simulink model "VD_L_filter"  (R2018b)
settings: Solver=ode8  StartTime=0.0  StopTime=1  RelTol=1e-3
undefined symbols (not defined in the file): C, L, Rn
libraries: powerlib x16, powerlib_meascontrol x8, peRmsMeasurement x4
settings Model: Creator=Anton  LastModifiedBy=VID Company
settings SFSimCC: SimUseLocalCustomCode=off
settings RTWCC: RTWUseLocalCustomCode=off
settings CodeAppCC: StateflowObjectComments=on
settings SimscapeCC: SimscapeNormalizeSystem=off

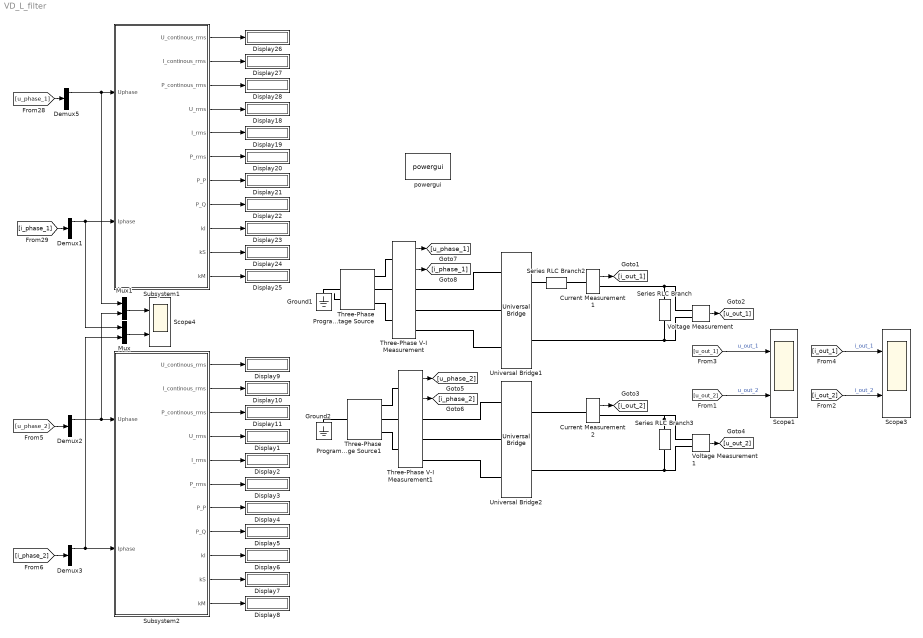
== system VD_L_filter ==
  Current Measurement1 : powerlib/Measurements/Current Measurement  PhasorSimulation=off  OutputType=Complex  PSBequivalent=0
  Current Measurement2 : powerlib/Measurements/Current Measurement  PhasorSimulation=off  OutputType=Complex  PSBequivalent=0
  Demux{1..3,5} (4 alike) : Demux  Outputs=3
  Display{1..11,18..28} (22 alike) : Display
  Ground1 : powerlib/Elements/Ground  LConnTagsString=a
  Ground2 : powerlib/Elements/Ground  LConnTagsString=a
  Mux : Mux  Inputs=2
  Mux1 : Mux  Inputs=2
  Scope1 : Scope  NumInputPorts=2
  Scope3 : Scope  NumInputPorts=2
  Scope4 : Scope  NumInputPorts=2
  Series RLC Branch : powerlib/Elements/Series RLC Branch  LConnTagsString=__new0  RConnTagsString=__new0  BranchType=R  Resistance=Rn  Inductance=250e-6  SetiL0=off  InitialCurrent=0  Capacitance=1e-6  Setx0=off  InitialVoltage=0  Measurements=None
  Series RLC Branch2 : powerlib/Elements/Series RLC Branch  LConnTagsString=__new0  RConnTagsString=__new0  BranchType=L  Resistance=1e-3  Inductance=L  SetiL0=off  InitialCurrent=0  Capacitance=C  Setx0=on  InitialVoltage=Un  Measurements=None
  Series RLC Branch3 : powerlib/Elements/Series RLC Branch  LConnTagsString=__new0  RConnTagsString=__new0  BranchType=R  Resistance=Rn  Inductance=250e-6  SetiL0=off  InitialCurrent=0  Capacitance=1e-6  Setx0=off  InitialVoltage=0  Measurements=None
  Subsystem1 : Subsystem
  Subsystem2 : Subsystem
  Three-Phase Programmable Voltage Source : powerlib/Electrical Sources/Three-Phase Programmable Voltage Source  PositiveSequence=[390 0 50]  VariationEntity=None  VariationType=Table of time-amplitude pairs  VariationTypeAlt=Step  VariationStep=0.5  VariationRate=10  VariationMagnitude=0.3  VariationFrequency=2  VariationTiming=[1 2]  VariationPhaseA=off  Amplitudes=[1 0.8 1.2 1.0]  TimeValues=[0 0.1 0.15 0.2]  HarmonicGeneration=off  HarmonicA=[3 0.2 -25 0]  HarmonicB=[2 0.15 35 2]  Timing="[0.05  3]"  BusType=swing  Pref=0  Qref=0  Qmin=-inf  Qmax=inf
  Three-Phase Programmable Voltage Source1 : powerlib/Electrical Sources/Three-Phase Programmable Voltage Source  PositiveSequence=[390 0 50]  VariationEntity=None  VariationType=Table of time-amplitude pairs  VariationTypeAlt=Step  VariationStep=0.5  VariationRate=10  VariationMagnitude=0.3  VariationFrequency=2  VariationTiming=[1 2]  VariationPhaseA=off  Amplitudes=[1 0.8 1.2 1.0]  TimeValues=[0 0.1 0.15 0.2]  HarmonicGeneration=off  HarmonicA=[3 0.2 -25 0]  HarmonicB=[2 0.15 35 2]  Timing="[0.05  3]"  BusType=swing  Pref=0  Qref=0  Qmin=-inf  Qmax=inf
  Three-Phase V-I Measurement : powerlib/Measurements/Three-Phase V-I Measurement  VoltageMeasurement=phase-to-ground  SetLabelV=off  LabelV=Vabc  Vpu=off  VpuLL=off  CurrentMeasurement=yes  SetLabelI=off  LabelI=Iabc  Ipu=off  Pbase=100e6  Vbase=500e3  OutputType=Complex  PhasorSimulation=off  PSBequivalent=0
  Three-Phase V-I Measurement1 : powerlib/Measurements/Three-Phase V-I Measurement  VoltageMeasurement=phase-to-ground  SetLabelV=off  LabelV=Vabc  Vpu=off  VpuLL=off  CurrentMeasurement=yes  SetLabelI=off  LabelI=Iabc  Ipu=off  Pbase=100e6  Vbase=500e3  OutputType=Complex  PhasorSimulation=off  PSBequivalent=0
  Universal Bridge1 : powerlib/Power Electronics/Universal Bridge  Arms=3  SnubberResistance=1e5  SnubberCapacitance=inf  Device=Diodes  Ron=1e-3  Lon=0  ForwardVoltages="[  0  0  ]"  ForwardVoltage=1  GTOparameters=[ 10e-6 , 20e-6 ]  IGBTparameters=[ 1e-6 , 2e-6 ]  Measurements=None  Measurements_2=None  converterType=Rectifier
  Universal Bridge2 : powerlib/Power Electronics/Universal Bridge  Arms=3  SnubberResistance=1e5  SnubberCapacitance=inf  Device=Diodes  Ron=1e-9  Lon=0  ForwardVoltages="[  0  0  ]"  ForwardVoltage=1  GTOparameters=[ 10e-6 , 20e-6 ]  IGBTparameters=[ 1e-6 , 2e-6 ]  Measurements=None  Measurements_2=None  converterType=Rectifier
  Voltage Measurement : powerlib/Measurements/Voltage Measurement  PhasorSimulation=off  OutputType=Complex  PSBequivalent=0
  Voltage Measurement1 : powerlib/Measurements/Voltage Measurement  PhasorSimulation=off  OutputType=Complex  PSBequivalent=0
  powergui : powerlib/powergui  Priority=1  SimulationMode=Discrete  SampleTime=1e-6  frequency=60  Iterations=50  frequencyindice=0  Pbase=100e6  ErrMax=1e-4  UnitsV=kV  UnitsW=MW  buscounter=0  FunctionMessages=off  echomessages=off  EnableUseOfTLC=off  CurrentSourceSwitches=off  DisableSnubberDevices=off  DisableRonSwitches=off  DisableVfSwitches=off  DisplayEquations=off  SolverType=Tustin/Backward Euler (TBE)  Interpol=off  ExternalGateDelay=off  methode=off  Ts=100  x0status=blocks  SPID=off  SwTol=0  HookPort=off  RestoreLinks=warning  ResistiveCurrentMeasurement=off  Frange=[0:2:500]  Ylog=off  Xlog=on  ShowGrid=off  save=off  variable=ZData  structure=0  ZoomFFT=off  StartTime=0.0  cycles=1  DisplayStyle=1  fundamental=60  FreqAxis=off  MaxFrequency=1000  frequencyindicesteady=1  RmsSteady=1  display=off
  wires:
  Three-Phase V-I Measurement/2 -> [i_phase_1]
  Three-Phase V-I Measurement/1 -> [u_phase_1]
  Voltage Measurement/1 -> [u_out_1]
  Current Measurement1/1 -> [i_out_1]
  Current Measurement2/1 -> [i_out_2]
  Voltage Measurement1/1 -> [u_out_2]
  [u_out_1] -> Scope1/1  "u_out_1"
  [u_out_2] -> Scope1/2  "u_out_2"
  [i_out_1] -> Scope3/1  "i_out_1"
  [i_out_2] -> Scope3/2  "i_out_2"
  Subsystem1/8(P_Q) -> Display22/1
  Subsystem1/2(I_continous_rms) -> Display27/1
  Subsystem1/7(P_P) -> Display21/1
  Subsystem1/4(U_rms) -> Display18/1
  Subsystem1/3(P_continous_rms) -> Display28/1
  Subsystem1/9(kI) -> Display23/1
  Subsystem1/11(kM) -> Display25/1
  Subsystem1/6(P_rms) -> Display20/1
  Subsystem1/10(kS) -> Display24/1
  Subsystem1/5(I_rms) -> Display19/1
  Subsystem1/1(U_continous_rms) -> Display26/1
  Three-Phase V-I Measurement1/1 -> [u_phase_2]
  Three-Phase V-I Measurement1/2 -> [i_phase_2]
  Mux/1 -> Scope4/2
  Mux1/1 -> Scope4/1
  [u_phase_1] -> Demux5/1
  Demux5/1 -> Mux1/1, Subsystem1/1(Uphase)
  [i_phase_1] -> Demux1/1
  Demux1/1 -> Mux/1, Subsystem1/2(Iphase)
  Subsystem2/10(kS) -> Display7/1
  Subsystem2/6(P_rms) -> Display3/1
  Subsystem2/1(U_continous_rms) -> Display9/1
  Subsystem2/5(I_rms) -> Display2/1
  Subsystem2/9(kI) -> Display6/1
  Subsystem2/4(U_rms) -> Display1/1
  Subsystem2/3(P_continous_rms) -> Display11/1
  Subsystem2/7(P_P) -> Display4/1
  Subsystem2/11(kM) -> Display8/1
  Subsystem2/2(I_continous_rms) -> Display10/1
  Subsystem2/8(P_Q) -> Display5/1
  Demux2/1 -> Mux1/2, Subsystem2/1(Uphase)
  [u_phase_2] -> Demux2/1
  Demux3/1 -> Mux/2, Subsystem2/2(Iphase)
  [i_phase_2] -> Demux3/1
  connections:
  Universal Bridge1/LConn1 -- Three-Phase V-I Measurement/RConn1
  Universal Bridge1/LConn3 -- Three-Phase V-I Measurement/RConn3
  Universal Bridge1/LConn2 -- Three-Phase V-I Measurement/RConn2
  Three-Phase Programmable Voltage Source/RConn1 -- Three-Phase V-I Measurement/LConn1
  Three-Phase Programmable Voltage Source/LConn1 -- Ground1/LConn1
  Three-Phase Programmable Voltage Source/RConn3 -- Three-Phase V-I Measurement/LConn3
  Three-Phase Programmable Voltage Source/RConn2 -- Three-Phase V-I Measurement/LConn2
  Series RLC Branch/RConn1 -- Universal Bridge1/RConn2 -- Voltage Measurement/LConn2
  Voltage Measurement/LConn1 -- Current Measurement1/RConn1 -- Series RLC Branch/LConn1
  Current Measurement1/LConn1 -- Series RLC Branch2/RConn1
  Voltage Measurement1/LConn2 -- Series RLC Branch3/RConn1 -- Universal Bridge2/RConn2
  Series RLC Branch3/LConn1 -- Voltage Measurement1/LConn1 -- Current Measurement2/RConn1
  Current Measurement2/LConn1 -- Universal Bridge2/RConn1
  Universal Bridge2/LConn2 -- Three-Phase V-I Measurement1/RConn2
  Three-Phase Programmable Voltage Source1/RConn3 -- Three-Phase V-I Measurement1/LConn3
  Three-Phase Programmable Voltage Source1/RConn1 -- Three-Phase V-I Measurement1/LConn1
  Three-Phase Programmable Voltage Source1/LConn1 -- Ground2/LConn1
  Three-Phase Programmable Voltage Source1/RConn2 -- Three-Phase V-I Measurement1/LConn2
  Universal Bridge2/LConn1 -- Three-Phase V-I Measurement1/RConn1
  Universal Bridge2/LConn3 -- Three-Phase V-I Measurement1/RConn3
  Series RLC Branch2/LConn1 -- Universal Bridge1/RConn1
  ?

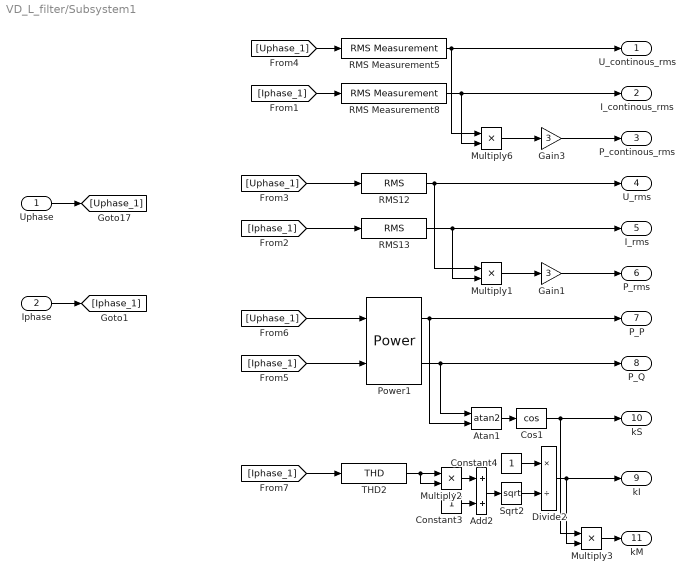
== system VD_L_filter/Subsystem1 ==
  Uphase : Inport
  Iphase : Inport  Port=2
  Add2 : Sum
  Atan1 : Trigonometry  Operator=atan2
  Constant3 : Constant
  Constant4 : Constant
  Cos1 : Trigonometry  Operator=cos
  Divide2 : Product  Inputs=*/
  Gain1 : Gain  Gain=3
  Gain3 : Gain  Gain=3
  Multiply{1..3,6} (4 alike) : Product
  Power1 : powerlib_meascontrol/Measurements/Power  Freq=50  Vinit=[1, 0]  Iinit=[1, 0]  Ts=0
      settings: SourceProductName=Simscape Power Systems
  RMS Measurement5 : peRmsMeasurement/RMS Measurement  LabelModeActiveChoice=Harmonic  F=50  SpecifyHarmonics=on  K=[1]  Ts=0
  RMS Measurement8 : peRmsMeasurement/RMS Measurement  LabelModeActiveChoice=Harmonic  F=50  SpecifyHarmonics=on  K=[1]  Ts=0
  RMS12 : powerlib_meascontrol/Measurements/RMS  TrueRMS=on  Freq=50  RMSInit=0  Ts=0
  RMS13 : powerlib_meascontrol/Measurements/RMS  TrueRMS=on  Freq=50  RMSInit=0  Ts=0
  Sqrt2 : Sqrt  SaturateOnIntegerOverflow=on
  THD2 : powerlib_meascontrol/Measurements/THD  Freq=50  Ts=0
  U_continous_rms : Outport
  I_continous_rms : Outport  Port=2
  P_continous_rms : Outport  Port=3
  U_rms : Outport  Port=4
  I_rms : Outport  Port=5
  P_rms : Outport  Port=6
  P_P : Outport  Port=7
  P_Q : Outport  Port=8
  kI : Outport  Port=9
  kS : Outport  Port=10
  kM : Outport  Port=11
  wires:
  RMS Measurement5/1 -> Multiply6/1, U_continous_rms/1
  RMS Measurement8/1 -> Multiply6/2, I_continous_rms/1
  [Uphase_1] -> RMS Measurement5/1
  [Iphase_1] -> RMS Measurement8/1
  Multiply6/1 -> Gain3/1
  RMS12/1 -> Multiply1/1, U_rms/1
  [Uphase_1] -> RMS12/1
  [Iphase_1] -> RMS13/1
  RMS13/1 -> Multiply1/2, I_rms/1
  Multiply1/1 -> Gain1/1
  Atan1/1 -> Cos1/1
  Power1/1 -> Atan1/2, P_P/1
  Power1/2 -> Atan1/1, P_Q/1
  [Uphase_1] -> Power1/1
  [Iphase_1] -> Power1/2
  Cos1/1 -> Multiply3/1, kS/1
  Sqrt2/1 -> Divide2/2
  THD2/1 -> Multiply2/1, Multiply2/2
  Constant3/1 -> Add2/2
  Multiply2/1 -> Add2/1
  Constant4/1 -> Divide2/1
  Divide2/1 -> Multiply3/2, kI/1
  Add2/1 -> Sqrt2/1
  [Iphase_1] -> THD2/1
  Multiply3/1 -> kM/1
  Gain3/1 -> P_continous_rms/1
  Gain1/1 -> P_rms/1
  Uphase/1 -> [Uphase_1]
  Iphase/1 -> [Iphase_1]

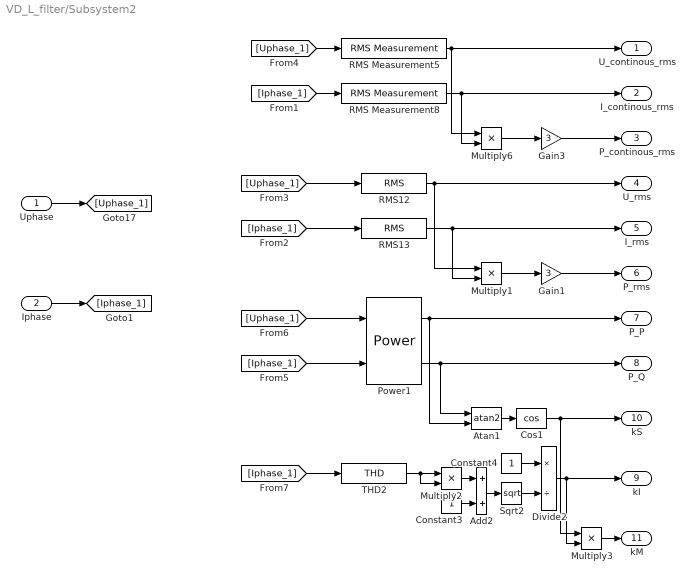
== system VD_L_filter/Subsystem2 ==
  Uphase : Inport
  Iphase : Inport  Port=2
  Add2 : Sum
  Atan1 : Trigonometry  Operator=atan2
  Constant3 : Constant
  Constant4 : Constant
  Cos1 : Trigonometry  Operator=cos
  Divide2 : Product  Inputs=*/
  Gain1 : Gain  Gain=3
  Gain3 : Gain  Gain=3
  Multiply{1..3,6} (4 alike) : Product
  Power1 : powerlib_meascontrol/Measurements/Power  Freq=50  Vinit=[1, 0]  Iinit=[1, 0]  Ts=0
      settings: SourceProductName=Simscape Power Systems
  RMS Measurement5 : peRmsMeasurement/RMS Measurement  LabelModeActiveChoice=Harmonic  F=50  SpecifyHarmonics=on  K=[1]  Ts=0
  RMS Measurement8 : peRmsMeasurement/RMS Measurement  LabelModeActiveChoice=Harmonic  F=50  SpecifyHarmonics=on  K=[1]  Ts=0
  RMS12 : powerlib_meascontrol/Measurements/RMS  TrueRMS=on  Freq=50  RMSInit=0  Ts=0
  RMS13 : powerlib_meascontrol/Measurements/RMS  TrueRMS=on  Freq=50  RMSInit=0  Ts=0
  Sqrt2 : Sqrt  SaturateOnIntegerOverflow=on
  THD2 : powerlib_meascontrol/Measurements/THD  Freq=50  Ts=0
  U_continous_rms : Outport
  I_continous_rms : Outport  Port=2
  P_continous_rms : Outport  Port=3
  U_rms : Outport  Port=4
  I_rms : Outport  Port=5
  P_rms : Outport  Port=6
  P_P : Outport  Port=7
  P_Q : Outport  Port=8
  kI : Outport  Port=9
  kS : Outport  Port=10
  kM : Outport  Port=11
  wires:
  RMS Measurement5/1 -> Multiply6/1, U_continous_rms/1
  RMS Measurement8/1 -> Multiply6/2, I_continous_rms/1
  [Uphase_1] -> RMS Measurement5/1
  [Iphase_1] -> RMS Measurement8/1
  Multiply6/1 -> Gain3/1
  RMS12/1 -> Multiply1/1, U_rms/1
  [Uphase_1] -> RMS12/1
  [Iphase_1] -> RMS13/1
  RMS13/1 -> Multiply1/2, I_rms/1
  Multiply1/1 -> Gain1/1
  Atan1/1 -> Cos1/1
  Power1/1 -> Atan1/2, P_P/1
  Power1/2 -> Atan1/1, P_Q/1
  [Uphase_1] -> Power1/1
  [Iphase_1] -> Power1/2
  Cos1/1 -> Multiply3/1, kS/1
  Sqrt2/1 -> Divide2/2
  THD2/1 -> Multiply2/1, Multiply2/2
  Constant3/1 -> Add2/2
  Multiply2/1 -> Add2/1
  Constant4/1 -> Divide2/1
  Divide2/1 -> Multiply3/2, kI/1
  Add2/1 -> Sqrt2/1
  [Iphase_1] -> THD2/1
  Multiply3/1 -> kM/1
  Gain3/1 -> P_continous_rms/1
  Gain1/1 -> P_rms/1
  Uphase/1 -> [Uphase_1]
  Iphase/1 -> [Iphase_1]
